simulink model "MotoreCC2"  (R2017a)
settings: Solver=VariableStepAuto  StartTime=0.0  StopTime=10.0  RelTol=1e-3
values from neighbouring files (symbols this model uses):
  b = 0.1    [MotoreCC.m]
  J = 0.01    [MotoreCC.m]
  K = 0.01    [MotoreCC.m]
  L = 0.5    [MotoreCC.m]
  R = 1    [MotoreCC.m]
settings Model: Creator=Michele  LastModifiedBy=Michele

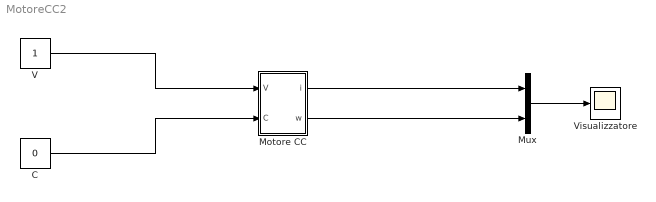
== system MotoreCC2 ==
  C : Constant  Value=0
  Motore CC : Subsystem
  Mux : Mux  Inputs=2
  V : Constant
  Visualizzatore : Scope
  wires:
  Mux/1 -> Visualizzatore/1
  V/1 -> Motore CC/1(V)
  C/1 -> Motore CC/2(C)
  Motore CC/1(i) -> Mux/1
  Motore CC/2(w) -> Mux/2

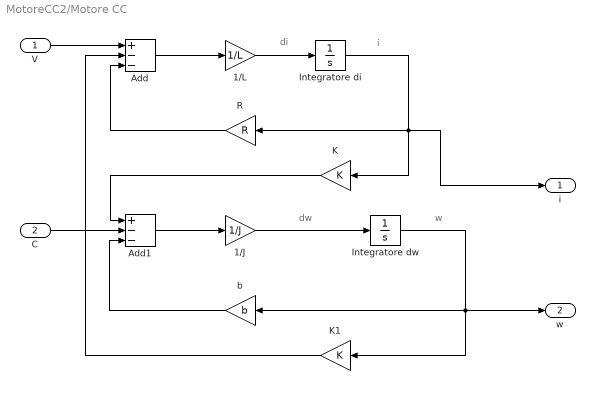
== system MotoreCC2/Motore CC ==
  note: w
  note: dw
  note: i
  note: di
  V : Inport
  C : Inport  Port=2
  1/J : Gain  Gain=1/J
  1/L : Gain  Gain=1/L
  Add : Sum  Inputs=+--
  Add1 : Sum  Inputs=+--
  Integratore di : Integrator
  Integratore dw : Integrator
  K : Gain  Gain=K
  K1 : Gain  Gain=K
  R : Gain  Gain=R
  b : Gain  Gain=b
  i : Outport
  w : Outport  Port=2
  wires:
  Add/1 -> 1/L/1
  Integratore di/1 -> i/1, K/1, R/1
  Integratore dw/1 -> w/1, K1/1, b/1
  1/L/1 -> Integratore di/1
  V/1 -> Add/1
  C/1 -> Add1/2
  Add1/1 -> 1/J/1
  1/J/1 -> Integratore dw/1
  R/1 -> Add/3
  K1/1 -> Add/2
  b/1 -> Add1/3
  K/1 -> Add1/1
